simulink model "lab2_circuit_model"  (R2025b)
settings: Solver=ode45  StartTime=0.0  StopTime=400  MaxStep=0.5  RelTol=1e-3
values from neighbouring files (symbols this model uses):
  A = 14.1208    [circuit_model.m]    (also in closed_sweep.m; controller_simualtion_result.m; open_loop.m)
  g_f1 = Rb/Ra    (= 0.0121951219512)    [circuit_model.m]
  g_p2 = (Rh/(Rg+Rh))*(1 + Rf2/Re)    (= 1)    [circuit_model.m]
  g_r1 = (Rd/(Rc+Rd))*(1 + Rb/Ra)    (= 0.0121951219512)    [circuit_model.m]
  ks = 0.6599    [circuit_model.m]    (also in closed_sweep.m; controller_simualtion_result.m; open_loop.m)
  r_m = 5    [circuit_model.m]    (also in closed_sweep.m; controller_simualtion_result.m)
  tau = 12.9898    [circuit_model.m]    (also in closed_sweep.m; controller_simualtion_result.m; open_loop.m)
  Vhover = 2.5    [circuit_model.m]    (also in closed_sweep.m; controller_simualtion_result.m; open_loop.m; velocity_position_plots.m)
  Vlev_out = levelOut(Rtrim)    [circuit_model.m]
  Voff1 = Vos1*(1 + Rb/Ra)    (= 0)    [circuit_model.m]
  Voff2 = Vos2*(1 + Rf2/Re)    (= 0)    [circuit_model.m]
  Vrail = 13.5    [circuit_model.m]
settings Model: Creator=MTMTAD006  LastModifiedBy=MTMTAD006

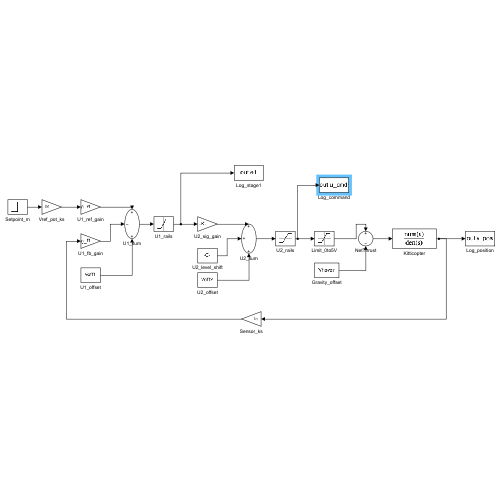
[thumbnail: Simulink's stored preview of the top-level diagram]
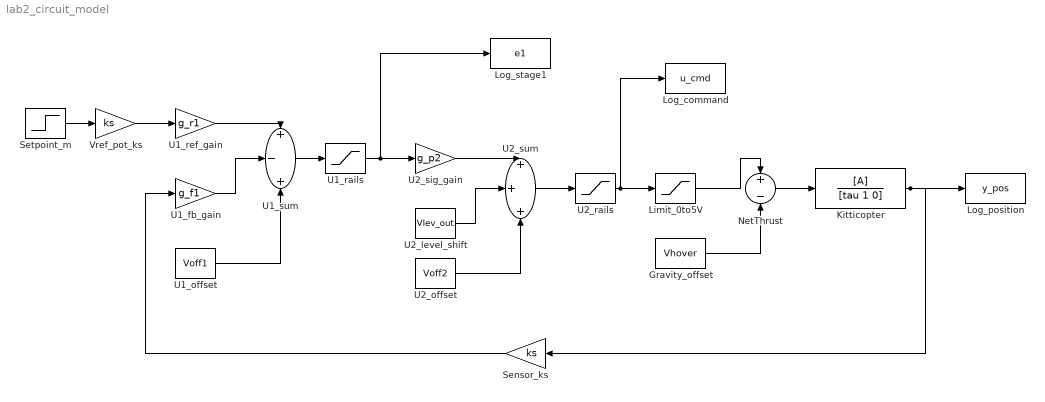
== system lab2_circuit_model ==
  Gravity_offset : Constant  Value=Vhover
  Kitticopter : TransferFcn  Numerator=[A]  Denominator=[tau 1 0]
  Limit_0to5V : Saturate  UpperLimit=5  LowerLimit=0
  Log_command : ToWorkspace  VariableName=u_cmd  SaveFormat=Timeseries  SampleTime=-1
  Log_position : ToWorkspace  VariableName=y_pos  SaveFormat=Timeseries  SampleTime=-1
  Log_stage1 : ToWorkspace  VariableName=e1  SaveFormat=Timeseries  SampleTime=-1
  NetThrust : Sum  Inputs=+-
  Sensor_ks : Gain  Gain=ks
  Setpoint_m : Step  Time=0  After=r_m  SampleTime=0
  U1_fb_gain : Gain  Gain=g_f1
  U1_offset : Constant  Value=Voff1
  U1_rails : Saturate  UpperLimit=Vrail  LowerLimit=-Vrail
  U1_ref_gain : Gain  Gain=g_r1
  U1_sum : Sum  Inputs=+-+
  U2_level_shift : Constant  Value=Vlev_out
  U2_offset : Constant  Value=Voff2
  U2_rails : Saturate  UpperLimit=Vrail  LowerLimit=-Vrail
  U2_sig_gain : Gain  Gain=g_p2
  U2_sum : Sum  Inputs=+++
  Vref_pot_ks : Gain  Gain=ks
  wires:
  Setpoint_m/1 -> Vref_pot_ks/1
  Vref_pot_ks/1 -> U1_ref_gain/1
  U1_ref_gain/1 -> U1_sum/1
  Sensor_ks/1 -> U1_fb_gain/1
  U1_fb_gain/1 -> U1_sum/2
  U1_offset/1 -> U1_sum/3
  U1_sum/1 -> U1_rails/1
  U1_rails/1 -> Log_stage1/1, U2_sig_gain/1
  U2_sig_gain/1 -> U2_sum/1
  U2_level_shift/1 -> U2_sum/2
  U2_offset/1 -> U2_sum/3
  U2_sum/1 -> U2_rails/1
  U2_rails/1 -> Log_command/1, Limit_0to5V/1
  Limit_0to5V/1 -> NetThrust/1
  Gravity_offset/1 -> NetThrust/2
  NetThrust/1 -> Kitticopter/1
  Kitticopter/1 -> Log_position/1, Sensor_ks/1
